simulink model "Robot"  (R2021a)
settings: Solver=FixedStepAuto  StartTime=0.0  StopTime=50.0  FixedStep=0.001  RelTol=1e-3  EnableMultiTasking=on
libraries: arduinolib x6, simulink x2
settings Model: SILPILModeSetting=veronly  ExtModeTrigDuration=2  Creator=drak0  LastModifiedBy=drak0
settings OptimizationCC: EnhancedBackFolding=on  PassReuseOutputArgsAs=Individual arguments  ZeroExternalMemoryAtStartup=off  ZeroInternalMemoryAtStartup=off  MaxStackSize=64  OptimizeBlockOrder=speed  DifferentSizesBufferReuse=on  OptimizationCustomize=off  EfficientTunableParamExpr=on
settings DebuggingCC: ParameterTunabilityLossMsg=error
settings HardwareCC: ProdBitPerInt=16  ProdBitPerPointer=16  ProdBitPerSizeT=16  ProdBitPerPtrDiffT=16  ProdLargestAtomicFloat=None  ProdWordSize=8  ProdHWDeviceType=Atmel->AVR  UseEmbeddedCoderFeatures=off  UseSimulinkCoderFeatures=off
settings SFSimCC: MATLABDynamicMemAlloc=off
settings RTWCC: SystemTargetFile=ert.tlc  HardwareBoard=Arduino Mega 2560  TemplateMakefile=ert_default_tmf  Toolchain=Arduino AVR  BuildConfiguration=Faster Runs
settings CodeAppCC: ForceParamTrailComments=on  IgnoreCustomStorageClasses=off  OperatorAnnotations=on  SimulinkDataObjDesc=on  SFDataObjDesc=on  InsertBlockDesc=on
settings ERTTargetCC: SupportContinuousTime=on  SupportNonInlinedSFcns=on  SupportVariableSizeSignals=on  ExtModeStaticAllocSize=2048

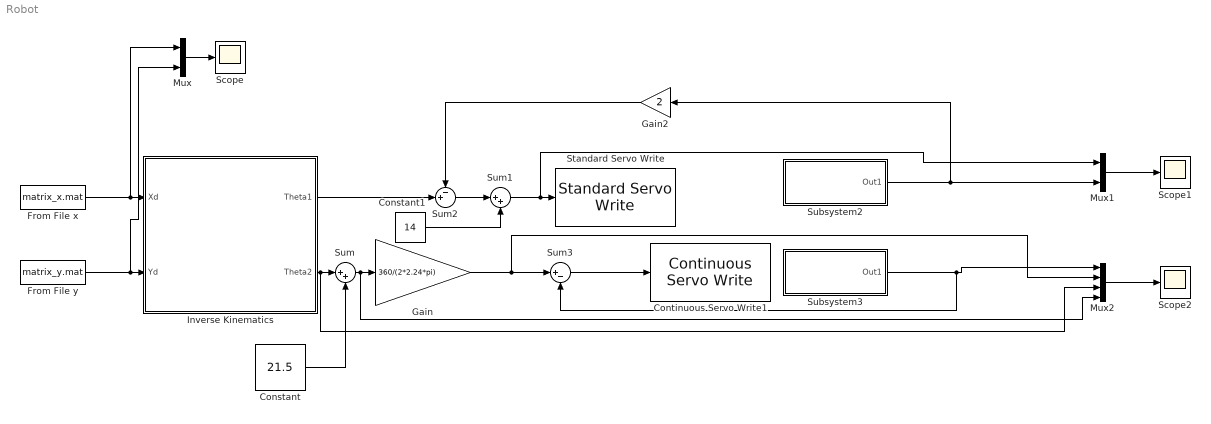
== system Robot ==
  Constant : Constant  Value=21.5
  Constant1 : Constant  Value=14
  Continuous Servo Write1 : arduinolib/Continuous Servo Write  pinNumber=11  ServoIndex=0  blockPlatform=ARDUINO
      settings: SourceProductBaseCode=ARDUINO
  From File x : FromFile  FileName=matrix_x.mat  SampleTime=0
  From File y : FromFile  FileName=matrix_y.mat  SampleTime=0
  Gain : Gain  Gain=360/(2*2.24*pi)
  Gain2 : Gain  Gain=2
  Inverse Kinematics : MATLAB Function  TreatAsAtomicUnit=on
  Mux : Mux  Inputs=2
  Mux1 : Mux  Inputs=2
  Mux2 : Mux
  Scope : Scope
  Scope1 : Scope
  Scope2 : Scope
  Standard Servo Write : arduinolib/Standard Servo Write  pinNumber=10  ServoIndex=1  blockPlatform=ARDUINO
  Subsystem2 : Subsystem
  Subsystem3 : Subsystem
  Sum : Sum  Inputs=|++
  Sum1 : Sum  Inputs=|++
  Sum2 : Sum  Inputs=-+|
  Sum3 : Sum  Inputs=|+-
  wires:
  Mux2/1 -> Scope2/1
  Subsystem3/1(Out1) -> Mux2/1, Sum3/2
  Sum3/1 -> Continuous Servo Write1/1
  Mux1/1 -> Scope1/1
  Subsystem2/1(Out1) -> Gain2/1, Mux1/2
  Mux/1 -> Scope/1
  Inverse Kinematics/1(Theta1) -> Sum2/2
  Gain/1 -> Mux2/2, Sum3/1
  Constant1/1 -> Sum1/2
  Sum1/1 -> Mux1/1, Standard Servo Write/1
  From File y/1 -> Mux/2, Inverse Kinematics/2(Yd)
  From File x/1 -> Mux/1, Inverse Kinematics/1(Xd)
  Inverse Kinematics/2(Theta2) -> Mux2/3, Sum/1
  Sum/1 -> Mux2/4, Gain/1
  Constant/1 -> Sum/2
  Sum2/1 -> Sum1/1
  Gain2/1 -> Sum2/1

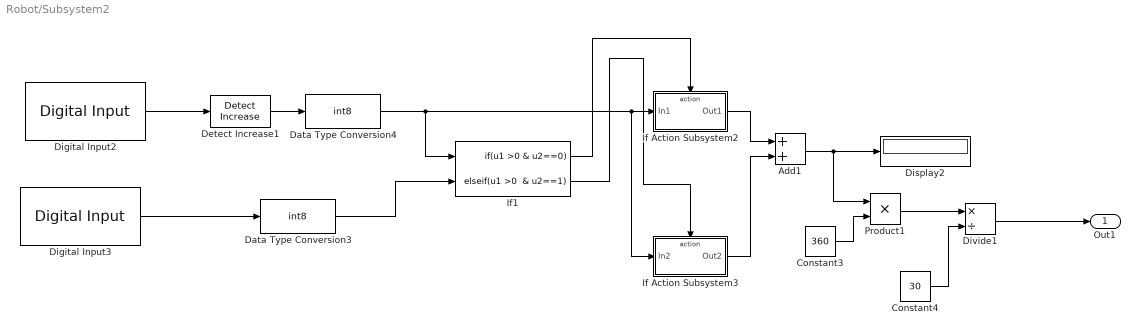
== system Robot/Subsystem2 ==
  Add1 : Sum
  Constant3 : Constant  Value=360
  Constant4 : Constant  Value=30
  Data Type Conversion3 : DataTypeConversion  OutDataTypeStr=int8
  Data Type Conversion4 : DataTypeConversion  OutDataTypeStr=int8
  Detect Increase1 : simulink/Logic and Bit Operations/Detect Increase  vinit=0.0  OutDataTypeStr=boolean
  Digital Input2 : arduinolib/Digital Input  pinNumber=2  mode=Default  Direction=input  SampleTime=-1  blockPlatform=arduino
  Digital Input3 : arduinolib/Digital Input  pinNumber=3  mode=Default  Direction=input  SampleTime=-1  blockPlatform=arduino
  Display2 : Display
  Divide1 : Product  Inputs=*/
  If Action Subsystem2 : Subsystem  TreatAsAtomicUnit=on
  If Action Subsystem3 : Subsystem  TreatAsAtomicUnit=on
  If1 : If  NumInputs=2  IfExpression=u1 >0 & u2==0  ElseIfExpressions="u1 >0  & u2==1"  ShowElse=off
  Product1 : Product
  Out1 : Outport
  wires:
  Divide1/1 -> Out1/1
  If Action Subsystem3/1(Out2) -> Add1/2
  Data Type Conversion4/1 -> If Action Subsystem3/1(In2), If Action Subsystem2/1(In1), If1/1
  If1/2 -> If Action Subsystem3/Action
  Constant3/1 -> Product1/2
  Add1/1 -> Product1/1, Display2/1
  Digital Input3/1 -> Data Type Conversion3/1
  Digital Input2/1 -> Detect Increase1/1
  If1/1 -> If Action Subsystem2/Action
  Data Type Conversion3/1 -> If1/2
  Constant4/1 -> Divide1/2
  Detect Increase1/1 -> Data Type Conversion4/1
  If Action Subsystem2/1(Out1) -> Add1/1
  Product1/1 -> Divide1/1

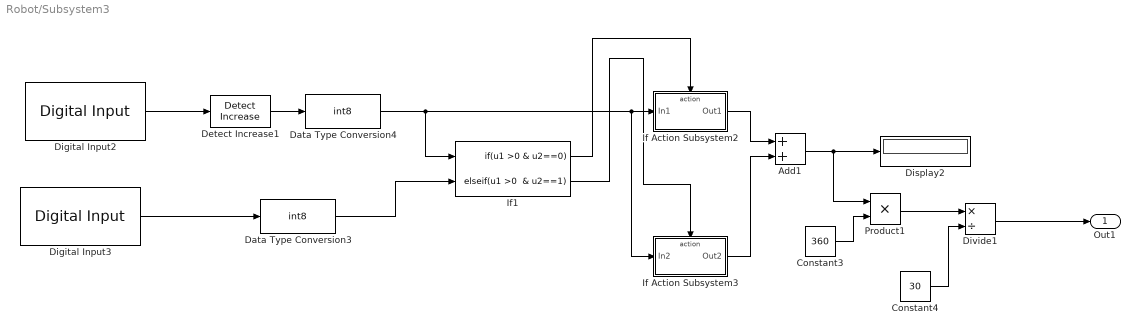
== system Robot/Subsystem3 ==
  Add1 : Sum
  Constant3 : Constant  Value=360
  Constant4 : Constant  Value=30
  Data Type Conversion3 : DataTypeConversion  OutDataTypeStr=int8
  Data Type Conversion4 : DataTypeConversion  OutDataTypeStr=int8
  Detect Increase1 : simulink/Logic and Bit Operations/Detect Increase  vinit=0.0  OutDataTypeStr=boolean
  Digital Input2 : arduinolib/Digital Input  pinNumber=4  mode=Default  Direction=input  SampleTime=-1  blockPlatform=arduino
  Digital Input3 : arduinolib/Digital Input  pinNumber=5  mode=Default  Direction=input  SampleTime=-1  blockPlatform=arduino
  Display2 : Display
  Divide1 : Product  Inputs=*/
  If Action Subsystem2 : Subsystem  TreatAsAtomicUnit=on
  If Action Subsystem3 : Subsystem  TreatAsAtomicUnit=on
  If1 : If  NumInputs=2  IfExpression=u1 >0 & u2==0  ElseIfExpressions="u1 >0  & u2==1"  ShowElse=off
  Product1 : Product
  Out1 : Outport
  wires:
  Divide1/1 -> Out1/1
  If Action Subsystem3/1(Out2) -> Add1/2
  Data Type Conversion4/1 -> If Action Subsystem3/1(In2), If Action Subsystem2/1(In1), If1/1
  If1/2 -> If Action Subsystem3/Action
  Constant3/1 -> Product1/2
  Add1/1 -> Product1/1, Display2/1
  Digital Input3/1 -> Data Type Conversion3/1
  Digital Input2/1 -> Detect Increase1/1
  If1/1 -> If Action Subsystem2/Action
  Data Type Conversion3/1 -> If1/2
  Constant4/1 -> Divide1/2
  Detect Increase1/1 -> Data Type Conversion4/1
  If Action Subsystem2/1(Out1) -> Add1/1
  Product1/1 -> Divide1/1

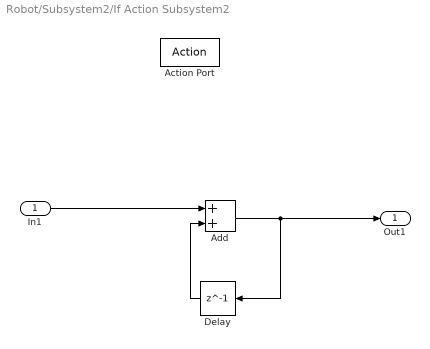
== system Robot/Subsystem2/If Action Subsystem2 ==
  In1 : Inport
  Action Port : ActionPort  ActionPortLabel=if(u1 >0 & u2==0)
  Add : Sum
  Delay : Delay  DelayLength=1  InitialCondition=0
  Out1 : Outport
  wires:
  In1/1 -> Add/1
  Add/1 -> Delay/1, Out1/1
  Delay/1 -> Add/2

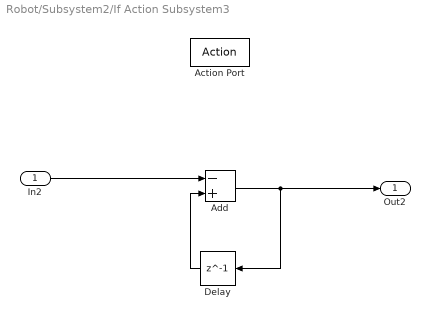
== system Robot/Subsystem2/If Action Subsystem3 ==
  In2 : Inport
  Action Port : ActionPort  ActionPortLabel="elseif( u1 >0  & u2==1)"
  Add : Sum  Inputs=-+
  Delay : Delay  DelayLength=1  InitialCondition=0
  Out2 : Outport
  wires:
  In2/1 -> Add/1
  Delay/1 -> Add/2
  Add/1 -> Delay/1, Out2/1

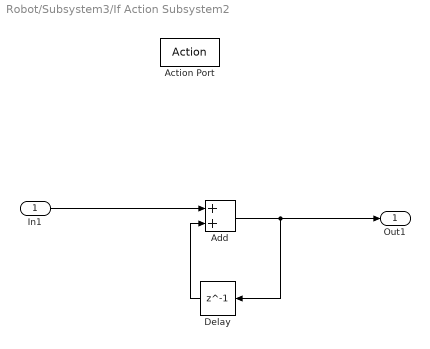
== system Robot/Subsystem3/If Action Subsystem2 ==
  In1 : Inport
  Action Port : ActionPort  ActionPortLabel=if(u1 >0 & u2==0)
  Add : Sum
  Delay : Delay  DelayLength=1  InitialCondition=0
  Out1 : Outport
  wires:
  In1/1 -> Add/1
  Add/1 -> Delay/1, Out1/1
  Delay/1 -> Add/2

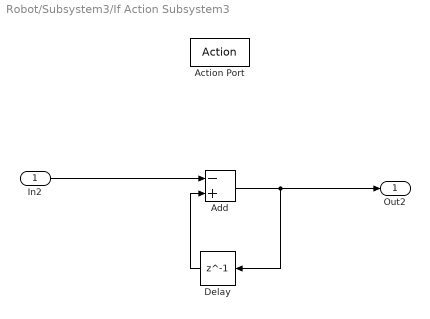
== system Robot/Subsystem3/If Action Subsystem3 ==
  In2 : Inport
  Action Port : ActionPort  ActionPortLabel="elseif( u1 >0  & u2==1)"
  Add : Sum  Inputs=-+
  Delay : Delay  DelayLength=1  InitialCondition=0
  Out2 : Outport
  wires:
  In2/1 -> Add/1
  Delay/1 -> Add/2
  Add/1 -> Delay/1, Out2/1

== matlab function Robot/Inverse Kinematics ==
  data: Xd input; Theta1 output; Yd input; Theta2 output
function [Theta1,Theta2] = InverseKinematics(Xd,Yd)
l1 = 2.25;
l2 = 21.5;
q1r = (atan2((sqrt(abs(-l1^2+Xd^2+Yd^2))+Yd),(l1+Xd)));
Theta1 = rad2deg(q1r);
Theta2 = -sin(q1r)*Xd +cos(q1r)*Yd-l2;
